simulink model "fullbridgesimple"  (R2016a)
settings: Solver=ode4  StartTime=0.0  StopTime=0.1  FixedStep=1e-6  RelTol=1e-3
settings Model: Creator=Heath  LastModifiedBy=rtw141
settings DataIOCC: LimitDataPoints=on  SaveFormat=Array  SignalLoggingSaveFormat=ModelDataLogs  SignalLoggingName=sigsOut
settings OptimizationCC: ExpressionDepthLimit=2147483647
settings DebuggingCC: SaveWithParameterizedLinksMsg=none  UnderspecifiedInitializationDetection=Classic  MergeDetectMultiDrivingBlocksExec=none  SignalResolutionControl=TryResolveAllWithWarning  MultiTaskDSMMsg=warning  MultiTaskCondExecSysMsg=none  StateNameClashWarn=warning  StrictBusMsg=None
settings HardwareCC: ProdBitPerPointer=32  ProdLargestAtomicFloat=None  ProdIntDivRoundTo=Undefined  ProdEndianess=Unspecified  ProdWordSize=32  ProdHWDeviceType=32-bit Generic  TargetUnknown=on
settings ModelReferenceCC: PropagateSignalLabelsOutOfModel=off
settings GRTTargetCC: CombineOutputUpdateFcns=off  GRTInterface=on
settings ConfigComp: CovModelRefEnable=Off

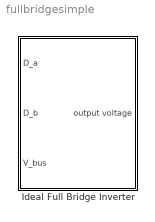
== system fullbridgesimple ==
  "Ideal Full Bridge Inverter " : Subsystem

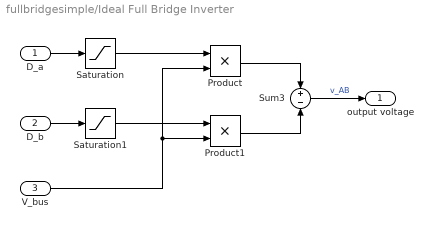
== system fullbridgesimple/Ideal Full Bridge Inverter  ==
  D_a : Inport
  D_b : Inport  Port=2
  V_bus : Inport  Port=3
  Product : Product
  Product1 : Product
  Saturation : Saturate  UpperLimit=1  LowerLimit=0
  Saturation1 : Saturate  UpperLimit=1  LowerLimit=0
  Sum3 : Sum  Inputs=+-  SaturateOnIntegerOverflow=on
  output voltage : Outport
  wires:
  Sum3/1 -> output voltage/1  "v_AB"
  D_a/1 -> Saturation/1
  D_b/1 -> Saturation1/1
  V_bus/1 -> Product1/2, Product/2
  Product/1 -> Sum3/1
  Product1/1 -> Sum3/2
  Saturation/1 -> Product/1
  Saturation1/1 -> Product1/1
